simulink model "Fehler_Provozierend"  (R2021a)
settings: Solver=VariableStepAuto  StartTime=0.0  StopTime=1  RelTol=1e-3
model workspace (MAT data in the model file):
  Kz = Simulink.Parameter
  Kz.Value = Simulink.data.Expression
  Kz.Value.ExpressionString = "(L/(Lc+ds))"
  Kz.DataType = 'auto'
  Kz.Dimensions = -1
  L = Simulink.Parameter
  L.Value = 52.8
  L.DataType = 'auto'
  L.Dimensions = [1 1]
  Lc = Simulink.Parameter
  Lc.Value = 4.4
  Lc.DataType = 'auto'
  Lc.Dimensions = [1 1]
  Rk = Simulink.Parameter
  Rk.Value = Simulink.data.Expression
  Rk.Value.ExpressionString = "Lc/v"
  Rk.DataType = 'auto'
  Rk.Dimensions = -1
  Tz = Simulink.Parameter
  Tz.Value = Simulink.data.Expression
  Tz.Value.ExpressionString = "L/v"
  Tz.DataType = 'auto'
  Tz.Dimensions = -1
  ds = Simulink.Parameter
  ds.Value = Simulink.data.Expression
  ds.Value.ExpressionString = "dt*v"
  ds.DataType = 'auto'
  ds.Dimensions = -1
  dt = Simulink.Parameter
  dt.Value = 1
  dt.DataType = 'auto'
  dt.Dimensions = [1 1]
  v = Simulink.Parameter
  v.Value = 13.89
  v.DataType = 'auto'
  v.Dimensions = [1 1]
libraries: EdgesLibrary x4, StreetLanesLibrary x3, SourcesAndSinksLibrary x2
settings Model: OrderedModelArguments=off  Creator=phill  LastModifiedBy=timyb
settings SolverCC: ZeroCrossAlgorithm=Adaptive

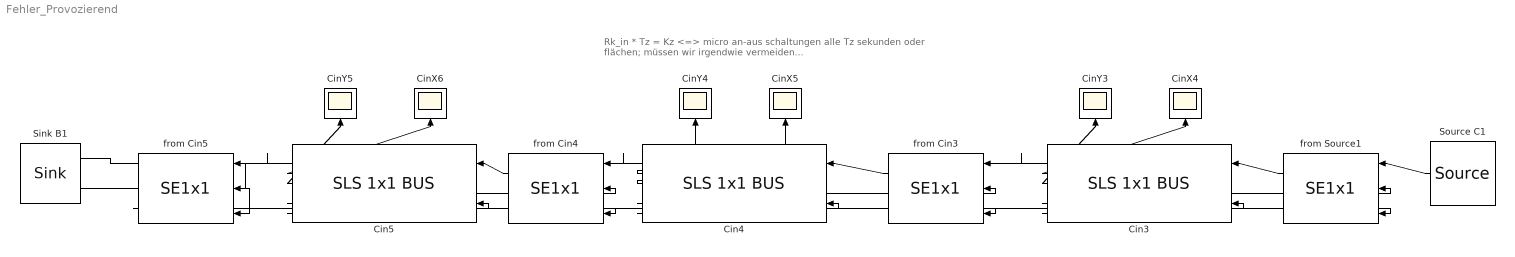
== system Fehler_Provozierend ==
  note: Rk_in * Tz = Kz   <=> micro an-aus schaltungen alle Tz sekunden
      | oder flächen; müssen wir irgendwie vermeiden...
  Cin3 : StreetLanesLibrary/SLS 1x1 BUS  Kz=2  Tz=2
  Cin4 : StreetLanesLibrary/SLS 1x1 BUS  Kz=2  Tz=2
  Cin5 : StreetLanesLibrary/SLS 1x1 BUS  Kz=2  Tz=2
  CinX4 : Scope
  CinX5 : Scope
  CinX6 : Scope
  CinY3 : Scope
  CinY4 : Scope
  CinY5 : Scope
  Sink B1 : SourcesAndSinksLibrary/Sink  SystemSampleTime=-1  VariantActivationTime=update diagram  Latency=0  AutoFrameSizeCalculation=off
      settings: PortSchema="{\"entries\":[{\"content\":{\"sides\":[{\"content\":{\"connectorIds\":[\"Out1\",\"Out2\"]},\"type\":\"ConnectorPlacement.EquallySpacedRectSide\",\"uuid\":\"9fd2383e-3590-4f0f-bafc-5a4adfbb32b4\"},{\"content\":{\"connectorIds\":[],\"side\":\"RIGHT\"},\"type\":\"ConnectorPlacement.EquallySpacedRectSide\",\"uuid\":\"1e687aa9-1098-45bd-a1f6-ea403f3f2897\"},{\"content\":{\"connectorIds\":[],\"side\":\"TOP\"},\"type\":\"ConnectorPlacement.EquallySpacedRectSide\",\"uuid\":\"fe6eaa71-085c-414b-983a-a0e72e52a49c\"}]},\"type\":\"ConnectorPlacement.EquallySpacedConnector\",\"uuid\":\"370c1712-4373-4726-99c2-6cb04807ece1\"}],\"packageUris\":[\"http://schema.mathworks.com/mf0/Connector/R2020b\"],\"version\":\"1.0\"}"
  Source C1 : SourcesAndSinksLibrary/Source  SystemSampleTime=-1  VariantActivationTime=update diagram  Latency=0  AutoFrameSizeCalculation=off
  from Cin3 : EdgesLibrary/SE1x1  Rk=1
  from Cin4 : EdgesLibrary/SE1x1  Rk=1
  from Cin5 : EdgesLibrary/SE1x1  Rk=1
  from Source1 : EdgesLibrary/SE1x1  Rk=1
  wires:
  Sink B1/1 -> from Cin5/2
  from Cin4/1 -> Cin5/1
  from Source1/1 -> Cin3/1
  Cin5/7 -> from Cin4/3
  Cin3/6 -> from Source1/2
  from Cin5/2 -> Cin5/2
  Cin5/6 -> from Cin4/2
  Cin5/4 -> CinY5/1
  Cin5/3 -> CinX6/1
  Cin5/2 -> from Cin5/1
  Source C1/1 -> from Source1/1
  Cin4/2 -> from Cin4/1
  Sink B1/2 -> from Cin5/3
  Cin4/7 -> from Cin3/3
  Cin3/2 -> from Cin3/1
  from Cin3/1 -> Cin4/1
  from Cin3/2 -> Cin3/2
  Cin4/6 -> from Cin3/2
  Cin4/4 -> CinY4/1
  Cin3/7 -> from Source1/3
  from Cin4/2 -> Cin4/2
  Cin3/3 -> CinX4/1
  Cin3/4 -> CinY3/1
  Cin4/3 -> CinX5/1
